simulink model "RLC"  (R2024a)
settings: Solver=VariableStepAuto  StartTime=0.0  StopTime=1e-3  MaxStep=1e-5  RelTol=1e-5
settings Model: Creator=perruquetti  LastModifiedBy=perruquetti

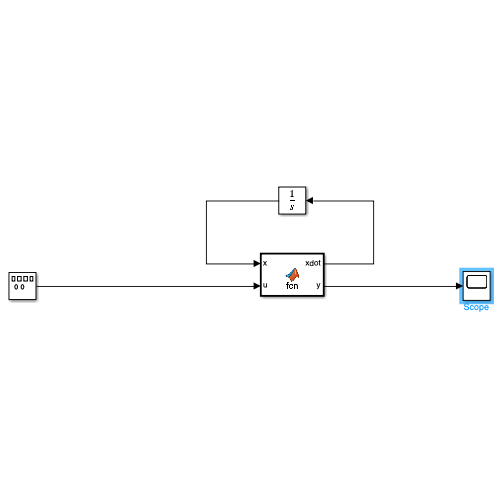
[thumbnail: Simulink's stored preview of the top-level diagram]
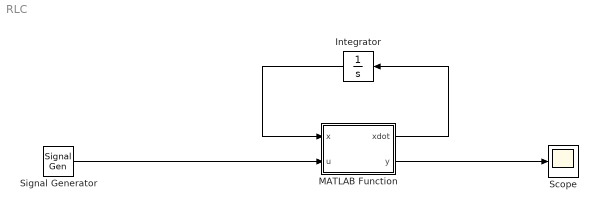
== system RLC ==
  Integrator : Integrator  InitialCondition="[2;  0.2]"
  MATLAB Function : MATLAB Function  TreatAsAtomicUnit=on
  Scope : Scope
  Signal Generator : SignalGenerator  Amplitude=10  Frequency=100  Units=rad/sec
  wires:
  MATLAB Function/1(xdot) -> Integrator/1
  Integrator/1 -> MATLAB Function/1(x)
  MATLAB Function/2(y) -> Scope/1
  Signal Generator/1 -> MATLAB Function/2(u)

== matlab function RLC/MATLAB Function ==
  data: x input; xdot output; u input; y output
function [xdot,y] = fcn(x,u)
%\frac{\mathrm {d}x_{1}}{\mathrm {d} t} (t)& =x_{2}(t),\nonumber\\
%\frac{\mathrm {d} x_{2}}{\mathrm {d} t}(t) & =-\omega_n^2 x_{1}(t)-2 \zeta \omega_n x_2(t).
%$\omega_n=\frac {1}{\sqrt{LC}}$ and $\zeta =\frac{R}{2} \sqrt{\frac{C}{L}}$.
% constants
    R = 10; 
    L = 1e-3;
    C = 1e-5;
    omega = 1/sqrt(L*C);
    zeta = R/2*sqrt(C/L);
% nonlinear set of equations
    xdot = [x(2);
        -omega*omega*x(1)-2*zeta*omega*x(2)];
    y = x';
